simulink model "untitled"  (R2019b)
settings: Solver=VariableStepAuto  StartTime=0.0  StopTime=10.0  RelTol=1e-3
libraries: simulink x1
settings Model: Creator=Mahban  LastModifiedBy=IwiLL
settings DebuggingCC: SFMachineParentedDataDiag=error  ArithmeticOperatorsInVariantConditions=warning
settings SFSimCC: CustomCodeUndefinedFunction=UseInterfaceOnly

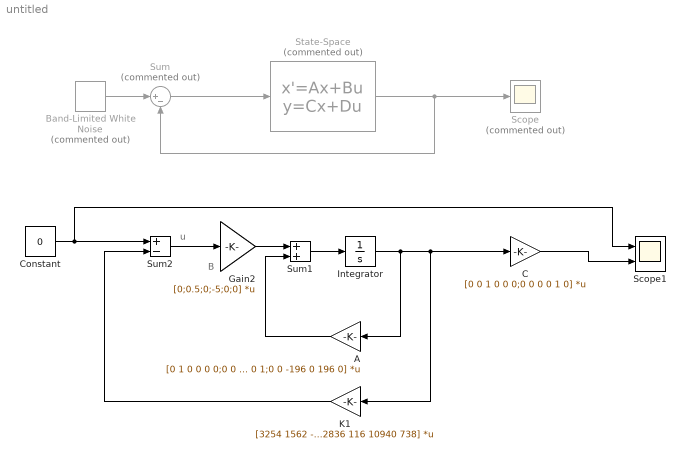
== system untitled ==
  note: u
  note: B
  A : Gain  Gain=[0 1 0 0 0 0;0 0 -0.98 0 0 0;0 0 0 1 0 0;0 0 205.8 0 -98 0;0 0 0 0 0 1;0 0 -196 0 196 0]  Multiplication=Matrix(K*u)
  Band-Limited White Noise : simulink/Sources/Band-Limited White Noise  Commented=on  Cov=[0.1]  Ts=0.1  seed=[23341]
  C : Gain  Gain=[0 0 1 0 0 0;0 0 0 0 1 0]  Multiplication=Matrix(K*u)
  Constant : Constant  Value=0
  Gain2 : Gain  Gain=[0;0.5;0;-5;0;0]  Multiplication=Matrix(K*u)
  Integrator : Integrator  InitialCondition=rand(6,1)
  K1 : Gain  Gain=[3254 1562 -2836 116 10940 738]  Multiplication=Matrix(K*u)
  Scope : Scope  Commented=on
  Scope1 : Scope  NumInputPorts=2
  State-Space : StateSpace  Commented=on  A=[0 1 0 0 0 0;0 0 -0.98 0 0 0;0 0 0 1 0 0;0 0 205.8 0 -98 0;0 0 0 0 0 1;0 0 -196 0 196 0]  B=[0;0.5;0;-5;0;0]  C=[0 0 1 0 0 0;0 0 0 0 1 0]  D=[0;0]  InitialCondition=0
  Sum : Sum  Commented=on  Inputs=|+-
  Sum1 : Sum
  Sum2 : Sum  Inputs=+-
  wires:
  Band-Limited White Noise/1 -> Sum/1
  Sum/1 -> State-Space/1
  State-Space/1 -> Scope/1, Sum/2
  Constant/1 -> Scope1/1, Sum2/1
  A/1 -> Sum1/2
  Sum2/1 -> Gain2/1
  Sum1/1 -> Integrator/1
  K1/1 -> Sum2/2
  Gain2/1 -> Sum1/1
  C/1 -> Scope1/2
  Integrator/1 -> A/1, C/1, K1/1
